simulink model "ROSCO"  (R2023a)
settings: Solver=ode4  StartTime=0.0  StopTime=TMax  FixedStep=simu.dt  RelTol=1e-3  EnableMultiTasking=on
undefined symbols (not defined in the file): A_total, Azimuth_list, B_total, Bd_total, C_total, D_total, Dd_total, DiscIntNeverNeededParam, F, n_FixFrameInputs, n_FixFrameOutputs, n_FixFrameStates2, n_RotTripletInputs, n_RotTripletOutputs, n_RotTripletStates2, new_seq_inp, new_seq_out, new_seq_states, OutList, Parameter, R, rpm2radps, simu, strmatch, uop_total, windspeed_list, wop_total, xop_total, yop_List_total
libraries: simulink x10
(part 3 of 5)

== system ROSCO/Monitor2/Cyclic Pitch controller/1P Cyclic Pitch Controller1/1P IPCDQ Filtering1/Moving 3P Notch Man Z/Moving 3P Filt Manual ==
  u : Inport
  rot speed (rad/s) : Inport  Port=2
  Den LPV : Subsystem
  Discrete Filter : DiscreteFilter  NumeratorSource=Input port  DenominatorSource=Input port  a0EqualsOne=on
      settings: InputPortMap=u0,p1,p3
  Num LPV : Subsystem
  Out1 : Outport  VectorParamsAs1DForOutWhenUnconnected=off
  wires:
  Den LPV/1(a) -> Discrete Filter/3
  rot speed (rad/s)/1 -> Num LPV/1(rot speed (rad/s)), Den LPV/1(rot speed (rad/s))
  Discrete Filter/1 -> Out1/1
  Num LPV/1(b) -> Discrete Filter/2
  u/1 -> Discrete Filter/1

== system ROSCO/Monitor2/Cyclic Pitch controller/1P Cyclic Pitch Controller1/1P IPCDQ Filtering1/Moving 6P Notch Man Y/Moving 6P Filt Manual ==
  u : Inport
  rot speed (rad/s) : Inport  Port=2
  Den LPV : Subsystem
  Discrete Filter : DiscreteFilter  NumeratorSource=Input port  DenominatorSource=Input port  a0EqualsOne=on
      settings: InputPortMap=u0,p1,p3
  Num LPV : Subsystem
  Out1 : Outport  VectorParamsAs1DForOutWhenUnconnected=off
  wires:
  Den LPV/1(a) -> Discrete Filter/3
  rot speed (rad/s)/1 -> Num LPV/1(rot speed (rad/s)), Den LPV/1(rot speed (rad/s))
  Discrete Filter/1 -> Out1/1
  Num LPV/1(b) -> Discrete Filter/2
  u/1 -> Discrete Filter/1

== system ROSCO/Monitor2/Cyclic Pitch controller/1P Cyclic Pitch Controller1/1P IPCDQ Filtering1/Moving 6P Notch Man Z/Moving 6P Filt Manual ==
  u : Inport
  rot speed (rad/s) : Inport  Port=2
  Den LPV : Subsystem
  Discrete Filter : DiscreteFilter  NumeratorSource=Input port  DenominatorSource=Input port  a0EqualsOne=on
      settings: InputPortMap=u0,p1,p3
  Num LPV : Subsystem
  Out1 : Outport  VectorParamsAs1DForOutWhenUnconnected=off
  wires:
  u/1 -> Discrete Filter/1
  Num LPV/1(b) -> Discrete Filter/2
  Discrete Filter/1 -> Out1/1
  rot speed (rad/s)/1 -> Den LPV/1(rot speed (rad/s)), Num LPV/1(rot speed (rad/s))
  Den LPV/1(a) -> Discrete Filter/3

== system ROSCO/Monitor2/Cyclic Pitch controller/1P Cyclic Pitch Controller1/M0 Signal Proc.1/Moving 1P Notch Man/Moving 1P Filt Manual ==
  u : Inport
  rot speed (rad/s) : Inport  Port=2
  Den LPV : Subsystem
  Discrete Filter : DiscreteFilter  NumeratorSource=Input port  DenominatorSource=Input port  a0EqualsOne=on
      settings: InputPortMap=u0,p1,p3
  Num LPV : Subsystem
  Out1 : Outport  VectorParamsAs1DForOutWhenUnconnected=off
  wires:
  Den LPV/1(a) -> Discrete Filter/3
  rot speed (rad/s)/1 -> Num LPV/1(rot speed (rad/s)), Den LPV/1(rot speed (rad/s))
  Discrete Filter/1 -> Out1/1
  Num LPV/1(b) -> Discrete Filter/2
  u/1 -> Discrete Filter/1

== system ROSCO/Monitor2/Cyclic Pitch controller/1P Cyclic Pitch Controller1/M0 Signal Proc.1/Moving 3P Notch Man/Moving 3P Filt Manual ==
  u : Inport
  rot speed (rad/s) : Inport  Port=2
  Den LPV : Subsystem
  Discrete Filter : DiscreteFilter  NumeratorSource=Input port  DenominatorSource=Input port  a0EqualsOne=on
      settings: InputPortMap=u0,p1,p3
  Num LPV : Subsystem
  Out1 : Outport  VectorParamsAs1DForOutWhenUnconnected=off
  wires:
  u/1 -> Discrete Filter/1
  Num LPV/1(b) -> Discrete Filter/2
  Discrete Filter/1 -> Out1/1
  rot speed (rad/s)/1 -> Den LPV/1(rot speed (rad/s)), Num LPV/1(rot speed (rad/s))
  Den LPV/1(a) -> Discrete Filter/3

== system ROSCO/Monitor2/Cyclic Pitch controller/2P Cyclic Pitch Controller2/1P IPCDQ Filtering1/Moving 3P Notch Man Y/Moving 3P Filt Manual ==
  u : Inport
  rot speed (rad/s) : Inport  Port=2
  Den LPV : Subsystem
  Discrete Filter : DiscreteFilter  NumeratorSource=Input port  DenominatorSource=Input port  a0EqualsOne=on
      settings: InputPortMap=u0,p1,p3
  Num LPV : Subsystem
  Out1 : Outport  VectorParamsAs1DForOutWhenUnconnected=off
  wires:
  u/1 -> Discrete Filter/1
  Num LPV/1(b) -> Discrete Filter/2
  Discrete Filter/1 -> Out1/1
  rot speed (rad/s)/1 -> Den LPV/1(rot speed (rad/s)), Num LPV/1(rot speed (rad/s))
  Den LPV/1(a) -> Discrete Filter/3

== system ROSCO/Monitor2/Cyclic Pitch controller/2P Cyclic Pitch Controller2/1P IPCDQ Filtering1/Moving 3P Notch Man Z/Moving 3P Filt Manual ==
  u : Inport
  rot speed (rad/s) : Inport  Port=2
  Den LPV : Subsystem
  Discrete Filter : DiscreteFilter  NumeratorSource=Input port  DenominatorSource=Input port  a0EqualsOne=on
      settings: InputPortMap=u0,p1,p3
  Num LPV : Subsystem
  Out1 : Outport  VectorParamsAs1DForOutWhenUnconnected=off
  wires:
  Den LPV/1(a) -> Discrete Filter/3
  rot speed (rad/s)/1 -> Num LPV/1(rot speed (rad/s)), Den LPV/1(rot speed (rad/s))
  Discrete Filter/1 -> Out1/1
  Num LPV/1(b) -> Discrete Filter/2
  u/1 -> Discrete Filter/1

== system ROSCO/Monitor2/Cyclic Pitch controller/2P Cyclic Pitch Controller2/1P IPCDQ Filtering1/Moving 6P Notch Man Y/Moving 6P Filt Manual ==
  u : Inport
  rot speed (rad/s) : Inport  Port=2
  Den LPV : Subsystem
  Discrete Filter : DiscreteFilter  NumeratorSource=Input port  DenominatorSource=Input port  a0EqualsOne=on
      settings: InputPortMap=u0,p1,p3
  Num LPV : Subsystem
  Out1 : Outport  VectorParamsAs1DForOutWhenUnconnected=off
  wires:
  Den LPV/1(a) -> Discrete Filter/3
  rot speed (rad/s)/1 -> Num LPV/1(rot speed (rad/s)), Den LPV/1(rot speed (rad/s))
  Discrete Filter/1 -> Out1/1
  Num LPV/1(b) -> Discrete Filter/2
  u/1 -> Discrete Filter/1

== system ROSCO/Monitor2/Cyclic Pitch controller/2P Cyclic Pitch Controller2/1P IPCDQ Filtering1/Moving 6P Notch Man Z/Moving 6P Filt Manual ==
  u : Inport
  rot speed (rad/s) : Inport  Port=2
  Den LPV : Subsystem
  Discrete Filter : DiscreteFilter  NumeratorSource=Input port  DenominatorSource=Input port  a0EqualsOne=on
      settings: InputPortMap=u0,p1,p3
  Num LPV : Subsystem
  Out1 : Outport  VectorParamsAs1DForOutWhenUnconnected=off
  wires:
  u/1 -> Discrete Filter/1
  Num LPV/1(b) -> Discrete Filter/2
  Discrete Filter/1 -> Out1/1
  rot speed (rad/s)/1 -> Den LPV/1(rot speed (rad/s)), Num LPV/1(rot speed (rad/s))
  Den LPV/1(a) -> Discrete Filter/3

== system ROSCO/Monitor2/Cyclic Pitch controller/2P Cyclic Pitch Controller2/M0 Signal Proc.1/Moving 1P Notch Man/Moving 1P Filt Manual ==
  u : Inport
  rot speed (rad/s) : Inport  Port=2
  Den LPV : Subsystem
  Discrete Filter : DiscreteFilter  NumeratorSource=Input port  DenominatorSource=Input port  a0EqualsOne=on
      settings: InputPortMap=u0,p1,p3
  Num LPV : Subsystem
  Out1 : Outport  VectorParamsAs1DForOutWhenUnconnected=off
  wires:
  Den LPV/1(a) -> Discrete Filter/3
  rot speed (rad/s)/1 -> Num LPV/1(rot speed (rad/s)), Den LPV/1(rot speed (rad/s))
  Discrete Filter/1 -> Out1/1
  Num LPV/1(b) -> Discrete Filter/2
  u/1 -> Discrete Filter/1

== system ROSCO/Monitor2/Cyclic Pitch controller/2P Cyclic Pitch Controller2/M0 Signal Proc.1/Moving 3P Notch Man/Moving 3P Filt Manual ==
  u : Inport
  rot speed (rad/s) : Inport  Port=2
  Den LPV : Subsystem
  Discrete Filter : DiscreteFilter  NumeratorSource=Input port  DenominatorSource=Input port  a0EqualsOne=on
      settings: InputPortMap=u0,p1,p3
  Num LPV : Subsystem
  Out1 : Outport  VectorParamsAs1DForOutWhenUnconnected=off
  wires:
  u/1 -> Discrete Filter/1
  Num LPV/1(b) -> Discrete Filter/2
  Discrete Filter/1 -> Out1/1
  rot speed (rad/s)/1 -> Den LPV/1(rot speed (rad/s)), Num LPV/1(rot speed (rad/s))
  Den LPV/1(a) -> Discrete Filter/3

== system ROSCO/Monitor2/Cyclic Pitch controller/1P Cyclic Pitch Controller1/1P IPCDQ Filtering1/Moving 3P Notch Man Y/Moving 3P Filt Manual/Den LPV ==
  rot speed (rad/s) : Inport
  1-D Lookup Table : Lookup_n-D  NumberOfTableDimensions=1  BreakpointsForDimension1=Parameter.Control.cIPC.PSM0_NF_3P.om_3P  BeginIndexSearchUsingPreviousIndexResult=on  Table=Parameter.Control.cIPC.PSM0_NF_3P.a_2  ExtrapMethod=Clip  InternalRulePriority=Speed  RndMeth=Simplest
  1-D Lookup Table1 : Lookup_n-D  NumberOfTableDimensions=1  BreakpointsForDimension1=Parameter.Control.cIPC.PSM0_NF_3P.om_3P  BeginIndexSearchUsingPreviousIndexResult=on  Table=Parameter.Control.cIPC.PSM0_NF_3P.a_1  ExtrapMethod=Clip  InternalRulePriority=Speed  RndMeth=Simplest
  1-D Lookup Table2 : Lookup_n-D  NumberOfTableDimensions=1  BreakpointsForDimension1=Parameter.Control.cIPC.PSM0_NF_3P.om_3P  BeginIndexSearchUsingPreviousIndexResult=on  Table=Parameter.Control.cIPC.PSM0_NF_3P.a_0  ExtrapMethod=Clip  InternalRulePriority=Speed  RndMeth=Simplest
  Mux : Mux  Inputs=3
  a : Outport  VectorParamsAs1DForOutWhenUnconnected=off
  wires:
  1-D Lookup Table/1 -> Mux/1
  1-D Lookup Table1/1 -> Mux/2
  Mux/1 -> a/1
  rot speed (rad/s)/1 -> 1-D Lookup Table2/1, 1-D Lookup Table/1, 1-D Lookup Table1/1
  1-D Lookup Table2/1 -> Mux/3

== system ROSCO/Monitor2/Cyclic Pitch controller/1P Cyclic Pitch Controller1/1P IPCDQ Filtering1/Moving 3P Notch Man Y/Moving 3P Filt Manual/Num LPV ==
  rot speed (rad/s) : Inport
  1-D Lookup Table : Lookup_n-D  NumberOfTableDimensions=1  BreakpointsForDimension1=Parameter.Control.cIPC.PSM0_NF_3P.om_3P  BeginIndexSearchUsingPreviousIndexResult=on  Table=Parameter.Control.cIPC.PSM0_NF_3P.b_2  ExtrapMethod=Clip  InternalRulePriority=Speed  RndMeth=Simplest
  1-D Lookup Table1 : Lookup_n-D  NumberOfTableDimensions=1  BreakpointsForDimension1=Parameter.Control.cIPC.PSM0_NF_3P.om_3P  BeginIndexSearchUsingPreviousIndexResult=on  Table=Parameter.Control.cIPC.PSM0_NF_3P.b_1  ExtrapMethod=Clip  InternalRulePriority=Speed  RndMeth=Simplest
  1-D Lookup Table2 : Lookup_n-D  NumberOfTableDimensions=1  BreakpointsForDimension1=Parameter.Control.cIPC.PSM0_NF_3P.om_3P  BeginIndexSearchUsingPreviousIndexResult=on  Table=Parameter.Control.cIPC.PSM0_NF_3P.b_0  ExtrapMethod=Clip  InternalRulePriority=Speed  RndMeth=Simplest
  Mux : Mux  Inputs=3
  b : Outport  VectorParamsAs1DForOutWhenUnconnected=off
  wires:
  1-D Lookup Table2/1 -> Mux/3
  rot speed (rad/s)/1 -> 1-D Lookup Table1/1, 1-D Lookup Table/1, 1-D Lookup Table2/1
  Mux/1 -> b/1
  1-D Lookup Table1/1 -> Mux/2
  1-D Lookup Table/1 -> Mux/1

== system ROSCO/Monitor2/Cyclic Pitch controller/1P Cyclic Pitch Controller1/1P IPCDQ Filtering1/Moving 3P Notch Man Z/Moving 3P Filt Manual/Den LPV ==
  rot speed (rad/s) : Inport
  1-D Lookup Table : Lookup_n-D  NumberOfTableDimensions=1  BreakpointsForDimension1=Parameter.Control.cIPC.PSM0_NF_3P.om_3P  BeginIndexSearchUsingPreviousIndexResult=on  Table=Parameter.Control.cIPC.PSM0_NF_3P.a_2  ExtrapMethod=Clip  InternalRulePriority=Speed  RndMeth=Simplest
  1-D Lookup Table1 : Lookup_n-D  NumberOfTableDimensions=1  BreakpointsForDimension1=Parameter.Control.cIPC.PSM0_NF_3P.om_3P  BeginIndexSearchUsingPreviousIndexResult=on  Table=Parameter.Control.cIPC.PSM0_NF_3P.a_1  ExtrapMethod=Clip  InternalRulePriority=Speed  RndMeth=Simplest
  1-D Lookup Table2 : Lookup_n-D  NumberOfTableDimensions=1  BreakpointsForDimension1=Parameter.Control.cIPC.PSM0_NF_3P.om_3P  BeginIndexSearchUsingPreviousIndexResult=on  Table=Parameter.Control.cIPC.PSM0_NF_3P.a_0  ExtrapMethod=Clip  InternalRulePriority=Speed  RndMeth=Simplest
  Mux : Mux  Inputs=3
  a : Outport  VectorParamsAs1DForOutWhenUnconnected=off
  wires:
  1-D Lookup Table2/1 -> Mux/3
  rot speed (rad/s)/1 -> 1-D Lookup Table1/1, 1-D Lookup Table/1, 1-D Lookup Table2/1
  Mux/1 -> a/1
  1-D Lookup Table1/1 -> Mux/2
  1-D Lookup Table/1 -> Mux/1

== system ROSCO/Monitor2/Cyclic Pitch controller/1P Cyclic Pitch Controller1/1P IPCDQ Filtering1/Moving 3P Notch Man Z/Moving 3P Filt Manual/Num LPV ==
  rot speed (rad/s) : Inport
  1-D Lookup Table : Lookup_n-D  NumberOfTableDimensions=1  BreakpointsForDimension1=Parameter.Control.cIPC.PSM0_NF_3P.om_3P  BeginIndexSearchUsingPreviousIndexResult=on  Table=Parameter.Control.cIPC.PSM0_NF_3P.b_2  ExtrapMethod=Clip  InternalRulePriority=Speed  RndMeth=Simplest
  1-D Lookup Table1 : Lookup_n-D  NumberOfTableDimensions=1  BreakpointsForDimension1=Parameter.Control.cIPC.PSM0_NF_3P.om_3P  BeginIndexSearchUsingPreviousIndexResult=on  Table=Parameter.Control.cIPC.PSM0_NF_3P.b_1  ExtrapMethod=Clip  InternalRulePriority=Speed  RndMeth=Simplest
  1-D Lookup Table2 : Lookup_n-D  NumberOfTableDimensions=1  BreakpointsForDimension1=Parameter.Control.cIPC.PSM0_NF_3P.om_3P  BeginIndexSearchUsingPreviousIndexResult=on  Table=Parameter.Control.cIPC.PSM0_NF_3P.b_0  ExtrapMethod=Clip  InternalRulePriority=Speed  RndMeth=Simplest
  Mux : Mux  Inputs=3
  b : Outport  VectorParamsAs1DForOutWhenUnconnected=off
  wires:
  1-D Lookup Table/1 -> Mux/1
  1-D Lookup Table1/1 -> Mux/2
  Mux/1 -> b/1
  rot speed (rad/s)/1 -> 1-D Lookup Table2/1, 1-D Lookup Table/1, 1-D Lookup Table1/1
  1-D Lookup Table2/1 -> Mux/3

== system ROSCO/Monitor2/Cyclic Pitch controller/1P Cyclic Pitch Controller1/1P IPCDQ Filtering1/Moving 6P Notch Man Y/Moving 6P Filt Manual/Den LPV ==
  rot speed (rad/s) : Inport
  1-D Lookup Table : Lookup_n-D  NumberOfTableDimensions=1  BreakpointsForDimension1=Parameter.Control.cIPC.PSM0_NF_6P.om_6P  BeginIndexSearchUsingPreviousIndexResult=on  Table=Parameter.Control.cIPC.PSM0_NF_6P.a_2  ExtrapMethod=Clip  InternalRulePriority=Speed  RndMeth=Simplest
  1-D Lookup Table1 : Lookup_n-D  NumberOfTableDimensions=1  BreakpointsForDimension1=Parameter.Control.cIPC.PSM0_NF_6P.om_6P  BeginIndexSearchUsingPreviousIndexResult=on  Table=Parameter.Control.cIPC.PSM0_NF_6P.a_1  ExtrapMethod=Clip  InternalRulePriority=Speed  RndMeth=Simplest
  1-D Lookup Table2 : Lookup_n-D  NumberOfTableDimensions=1  BreakpointsForDimension1=Parameter.Control.cIPC.PSM0_NF_6P.om_6P  BeginIndexSearchUsingPreviousIndexResult=on  Table=Parameter.Control.cIPC.PSM0_NF_6P.a_0  ExtrapMethod=Clip  InternalRulePriority=Speed  RndMeth=Simplest
  Mux : Mux  Inputs=3
  a : Outport  VectorParamsAs1DForOutWhenUnconnected=off
  wires:
  1-D Lookup Table2/1 -> Mux/3
  rot speed (rad/s)/1 -> 1-D Lookup Table1/1, 1-D Lookup Table/1, 1-D Lookup Table2/1
  Mux/1 -> a/1
  1-D Lookup Table1/1 -> Mux/2
  1-D Lookup Table/1 -> Mux/1

== system ROSCO/Monitor2/Cyclic Pitch controller/1P Cyclic Pitch Controller1/1P IPCDQ Filtering1/Moving 6P Notch Man Y/Moving 6P Filt Manual/Num LPV ==
  rot speed (rad/s) : Inport
  1-D Lookup Table : Lookup_n-D  NumberOfTableDimensions=1  BreakpointsForDimension1=Parameter.Control.cIPC.PSM0_NF_6P.om_6P  BeginIndexSearchUsingPreviousIndexResult=on  Table=Parameter.Control.cIPC.PSM0_NF_6P.b_2  ExtrapMethod=Clip  InternalRulePriority=Speed  RndMeth=Simplest
  1-D Lookup Table1 : Lookup_n-D  NumberOfTableDimensions=1  BreakpointsForDimension1=Parameter.Control.cIPC.PSM0_NF_6P.om_6P  BeginIndexSearchUsingPreviousIndexResult=on  Table=Parameter.Control.cIPC.PSM0_NF_6P.b_1  ExtrapMethod=Clip  InternalRulePriority=Speed  RndMeth=Simplest
  1-D Lookup Table2 : Lookup_n-D  NumberOfTableDimensions=1  BreakpointsForDimension1=Parameter.Control.cIPC.PSM0_NF_6P.om_6P  BeginIndexSearchUsingPreviousIndexResult=on  Table=Parameter.Control.cIPC.PSM0_NF_6P.b_0  ExtrapMethod=Clip  InternalRulePriority=Speed  RndMeth=Simplest
  Mux : Mux  Inputs=3
  b : Outport  VectorParamsAs1DForOutWhenUnconnected=off
  wires:
  1-D Lookup Table/1 -> Mux/1
  1-D Lookup Table1/1 -> Mux/2
  Mux/1 -> b/1
  rot speed (rad/s)/1 -> 1-D Lookup Table2/1, 1-D Lookup Table1/1, 1-D Lookup Table/1
  1-D Lookup Table2/1 -> Mux/3

== system ROSCO/Monitor2/Cyclic Pitch controller/1P Cyclic Pitch Controller1/1P IPCDQ Filtering1/Moving 6P Notch Man Z/Moving 6P Filt Manual/Den LPV ==
  rot speed (rad/s) : Inport
  1-D Lookup Table : Lookup_n-D  NumberOfTableDimensions=1  BreakpointsForDimension1=Parameter.Control.cIPC.PSM0_NF_6P.om_6P  BeginIndexSearchUsingPreviousIndexResult=on  Table=Parameter.Control.cIPC.PSM0_NF_6P.a_2  ExtrapMethod=Clip  InternalRulePriority=Speed  RndMeth=Simplest
  1-D Lookup Table1 : Lookup_n-D  NumberOfTableDimensions=1  BreakpointsForDimension1=Parameter.Control.cIPC.PSM0_NF_6P.om_6P  BeginIndexSearchUsingPreviousIndexResult=on  Table=Parameter.Control.cIPC.PSM0_NF_6P.a_1  ExtrapMethod=Clip  InternalRulePriority=Speed  RndMeth=Simplest
  1-D Lookup Table2 : Lookup_n-D  NumberOfTableDimensions=1  BreakpointsForDimension1=Parameter.Control.cIPC.PSM0_NF_6P.om_6P  BeginIndexSearchUsingPreviousIndexResult=on  Table=Parameter.Control.cIPC.PSM0_NF_6P.a_0  ExtrapMethod=Clip  InternalRulePriority=Speed  RndMeth=Simplest
  Mux : Mux  Inputs=3
  a : Outport  VectorParamsAs1DForOutWhenUnconnected=off
  wires:
  1-D Lookup Table/1 -> Mux/1
  1-D Lookup Table1/1 -> Mux/2
  Mux/1 -> a/1
  rot speed (rad/s)/1 -> 1-D Lookup Table2/1, 1-D Lookup Table/1, 1-D Lookup Table1/1
  1-D Lookup Table2/1 -> Mux/3

== system ROSCO/Monitor2/Cyclic Pitch controller/1P Cyclic Pitch Controller1/1P IPCDQ Filtering1/Moving 6P Notch Man Z/Moving 6P Filt Manual/Num LPV ==
  rot speed (rad/s) : Inport
  1-D Lookup Table : Lookup_n-D  NumberOfTableDimensions=1  BreakpointsForDimension1=Parameter.Control.cIPC.PSM0_NF_6P.om_6P  BeginIndexSearchUsingPreviousIndexResult=on  Table=Parameter.Control.cIPC.PSM0_NF_6P.b_2  ExtrapMethod=Clip  InternalRulePriority=Speed  RndMeth=Simplest
  1-D Lookup Table1 : Lookup_n-D  NumberOfTableDimensions=1  BreakpointsForDimension1=Parameter.Control.cIPC.PSM0_NF_6P.om_6P  BeginIndexSearchUsingPreviousIndexResult=on  Table=Parameter.Control.cIPC.PSM0_NF_6P.b_1  ExtrapMethod=Clip  InternalRulePriority=Speed  RndMeth=Simplest
  1-D Lookup Table2 : Lookup_n-D  NumberOfTableDimensions=1  BreakpointsForDimension1=Parameter.Control.cIPC.PSM0_NF_6P.om_6P  BeginIndexSearchUsingPreviousIndexResult=on  Table=Parameter.Control.cIPC.PSM0_NF_6P.b_0  ExtrapMethod=Clip  InternalRulePriority=Speed  RndMeth=Simplest
  Mux : Mux  Inputs=3
  b : Outport  VectorParamsAs1DForOutWhenUnconnected=off
  wires:
  1-D Lookup Table2/1 -> Mux/3
  rot speed (rad/s)/1 -> 1-D Lookup Table1/1, 1-D Lookup Table/1, 1-D Lookup Table2/1
  Mux/1 -> b/1
  1-D Lookup Table1/1 -> Mux/2
  1-D Lookup Table/1 -> Mux/1

== system ROSCO/Monitor2/Cyclic Pitch controller/1P Cyclic Pitch Controller1/M0 Signal Proc.1/Moving 1P Notch Man/Moving 1P Filt Manual/Den LPV ==
  rot speed (rad/s) : Inport
  1-D Lookup Table : Lookup_n-D  NumberOfTableDimensions=1  BreakpointsForDimension1=Parameter.Control.cIPC.PSM0_NF_1P.om_1P  BeginIndexSearchUsingPreviousIndexResult=on  Table=Parameter.Control.cIPC.PSM0_NF_1P.a_2  ExtrapMethod=Clip  InternalRulePriority=Speed  RndMeth=Simplest
  1-D Lookup Table1 : Lookup_n-D  NumberOfTableDimensions=1  BreakpointsForDimension1=Parameter.Control.cIPC.PSM0_NF_1P.om_1P  BeginIndexSearchUsingPreviousIndexResult=on  Table=Parameter.Control.cIPC.PSM0_NF_1P.a_1  ExtrapMethod=Clip  InternalRulePriority=Speed  RndMeth=Simplest
  1-D Lookup Table2 : Lookup_n-D  NumberOfTableDimensions=1  BreakpointsForDimension1=Parameter.Control.cIPC.PSM0_NF_1P.om_1P  BeginIndexSearchUsingPreviousIndexResult=on  Table=Parameter.Control.cIPC.PSM0_NF_1P.a_0  ExtrapMethod=Clip  InternalRulePriority=Speed  RndMeth=Simplest
  Mux : Mux  Inputs=3
  a : Outport  VectorParamsAs1DForOutWhenUnconnected=off
  wires:
  1-D Lookup Table2/1 -> Mux/3
  rot speed (rad/s)/1 -> 1-D Lookup Table1/1, 1-D Lookup Table/1, 1-D Lookup Table2/1
  Mux/1 -> a/1
  1-D Lookup Table1/1 -> Mux/2
  1-D Lookup Table/1 -> Mux/1

== system ROSCO/Monitor2/Cyclic Pitch controller/1P Cyclic Pitch Controller1/M0 Signal Proc.1/Moving 1P Notch Man/Moving 1P Filt Manual/Num LPV ==
  rot speed (rad/s) : Inport
  1-D Lookup Table : Lookup_n-D  NumberOfTableDimensions=1  BreakpointsForDimension1=Parameter.Control.cIPC.PSM0_NF_1P.om_1P  BeginIndexSearchUsingPreviousIndexResult=on  Table=Parameter.Control.cIPC.PSM0_NF_1P.b_2  ExtrapMethod=Clip  InternalRulePriority=Speed  RndMeth=Simplest
  1-D Lookup Table1 : Lookup_n-D  NumberOfTableDimensions=1  BreakpointsForDimension1=Parameter.Control.cIPC.PSM0_NF_1P.om_1P  BeginIndexSearchUsingPreviousIndexResult=on  Table=Parameter.Control.cIPC.PSM0_NF_1P.b_1  ExtrapMethod=Clip  InternalRulePriority=Speed  RndMeth=Simplest
  1-D Lookup Table2 : Lookup_n-D  NumberOfTableDimensions=1  BreakpointsForDimension1=Parameter.Control.cIPC.PSM0_NF_1P.om_1P  BeginIndexSearchUsingPreviousIndexResult=on  Table=Parameter.Control.cIPC.PSM0_NF_1P.b_0  ExtrapMethod=Clip  InternalRulePriority=Speed  RndMeth=Simplest
  Mux : Mux  Inputs=3
  b : Outport  VectorParamsAs1DForOutWhenUnconnected=off
  wires:
  1-D Lookup Table/1 -> Mux/1
  1-D Lookup Table1/1 -> Mux/2
  Mux/1 -> b/1
  rot speed (rad/s)/1 -> 1-D Lookup Table2/1, 1-D Lookup Table/1, 1-D Lookup Table1/1
  1-D Lookup Table2/1 -> Mux/3

== system ROSCO/Monitor2/Cyclic Pitch controller/1P Cyclic Pitch Controller1/M0 Signal Proc.1/Moving 3P Notch Man/Moving 3P Filt Manual/Den LPV ==
  rot speed (rad/s) : Inport
  1-D Lookup Table : Lookup_n-D  NumberOfTableDimensions=1  BreakpointsForDimension1=Parameter.Control.cIPC.PSM0_NF_3P.om_3P  BeginIndexSearchUsingPreviousIndexResult=on  Table=Parameter.Control.cIPC.PSM0_NF_3P.a_2  ExtrapMethod=Clip  InternalRulePriority=Speed  RndMeth=Simplest
  1-D Lookup Table1 : Lookup_n-D  NumberOfTableDimensions=1  BreakpointsForDimension1=Parameter.Control.cIPC.PSM0_NF_3P.om_3P  BeginIndexSearchUsingPreviousIndexResult=on  Table=Parameter.Control.cIPC.PSM0_NF_3P.a_1  ExtrapMethod=Clip  InternalRulePriority=Speed  RndMeth=Simplest
  1-D Lookup Table2 : Lookup_n-D  NumberOfTableDimensions=1  BreakpointsForDimension1=Parameter.Control.cIPC.PSM0_NF_3P.om_3P  BeginIndexSearchUsingPreviousIndexResult=on  Table=Parameter.Control.cIPC.PSM0_NF_3P.a_0  ExtrapMethod=Clip  InternalRulePriority=Speed  RndMeth=Simplest
  Mux : Mux  Inputs=3
  a : Outport  VectorParamsAs1DForOutWhenUnconnected=off
  wires:
  1-D Lookup Table/1 -> Mux/1
  1-D Lookup Table1/1 -> Mux/2
  Mux/1 -> a/1
  rot speed (rad/s)/1 -> 1-D Lookup Table2/1, 1-D Lookup Table/1, 1-D Lookup Table1/1
  1-D Lookup Table2/1 -> Mux/3

== system ROSCO/Monitor2/Cyclic Pitch controller/1P Cyclic Pitch Controller1/M0 Signal Proc.1/Moving 3P Notch Man/Moving 3P Filt Manual/Num LPV ==
  rot speed (rad/s) : Inport
  1-D Lookup Table : Lookup_n-D  NumberOfTableDimensions=1  BreakpointsForDimension1=Parameter.Control.cIPC.PSM0_NF_3P.om_3P  BeginIndexSearchUsingPreviousIndexResult=on  Table=Parameter.Control.cIPC.PSM0_NF_3P.b_2  ExtrapMethod=Clip  InternalRulePriority=Speed  RndMeth=Simplest
  1-D Lookup Table1 : Lookup_n-D  NumberOfTableDimensions=1  BreakpointsForDimension1=Parameter.Control.cIPC.PSM0_NF_3P.om_3P  BeginIndexSearchUsingPreviousIndexResult=on  Table=Parameter.Control.cIPC.PSM0_NF_3P.b_1  ExtrapMethod=Clip  InternalRulePriority=Speed  RndMeth=Simplest
  1-D Lookup Table2 : Lookup_n-D  NumberOfTableDimensions=1  BreakpointsForDimension1=Parameter.Control.cIPC.PSM0_NF_3P.om_3P  BeginIndexSearchUsingPreviousIndexResult=on  Table=Parameter.Control.cIPC.PSM0_NF_3P.b_0  ExtrapMethod=Clip  InternalRulePriority=Speed  RndMeth=Simplest
  Mux : Mux  Inputs=3
  b : Outport  VectorParamsAs1DForOutWhenUnconnected=off
  wires:
  1-D Lookup Table2/1 -> Mux/3
  rot speed (rad/s)/1 -> 1-D Lookup Table1/1, 1-D Lookup Table/1, 1-D Lookup Table2/1
  Mux/1 -> b/1
  1-D Lookup Table1/1 -> Mux/2
  1-D Lookup Table/1 -> Mux/1

== system ROSCO/Monitor2/Cyclic Pitch controller/2P Cyclic Pitch Controller2/1P IPCDQ Filtering1/Moving 3P Notch Man Y/Moving 3P Filt Manual/Den LPV ==
  rot speed (rad/s) : Inport
  1-D Lookup Table : Lookup_n-D  NumberOfTableDimensions=1  BreakpointsForDimension1=Parameter.Control.cIPC.PSM0_NF_3P.om_3P  BeginIndexSearchUsingPreviousIndexResult=on  Table=Parameter.Control.cIPC.PSM0_NF_3P.a_2  ExtrapMethod=Clip  InternalRulePriority=Speed  RndMeth=Simplest
  1-D Lookup Table1 : Lookup_n-D  NumberOfTableDimensions=1  BreakpointsForDimension1=Parameter.Control.cIPC.PSM0_NF_3P.om_3P  BeginIndexSearchUsingPreviousIndexResult=on  Table=Parameter.Control.cIPC.PSM0_NF_3P.a_1  ExtrapMethod=Clip  InternalRulePriority=Speed  RndMeth=Simplest
  1-D Lookup Table2 : Lookup_n-D  NumberOfTableDimensions=1  BreakpointsForDimension1=Parameter.Control.cIPC.PSM0_NF_3P.om_3P  BeginIndexSearchUsingPreviousIndexResult=on  Table=Parameter.Control.cIPC.PSM0_NF_3P.a_0  ExtrapMethod=Clip  InternalRulePriority=Speed  RndMeth=Simplest
  Mux : Mux  Inputs=3
  a : Outport  VectorParamsAs1DForOutWhenUnconnected=off
  wires:
  1-D Lookup Table/1 -> Mux/1
  1-D Lookup Table1/1 -> Mux/2
  Mux/1 -> a/1
  rot speed (rad/s)/1 -> 1-D Lookup Table2/1, 1-D Lookup Table/1, 1-D Lookup Table1/1
  1-D Lookup Table2/1 -> Mux/3

== system ROSCO/Monitor2/Cyclic Pitch controller/2P Cyclic Pitch Controller2/1P IPCDQ Filtering1/Moving 3P Notch Man Y/Moving 3P Filt Manual/Num LPV ==
  rot speed (rad/s) : Inport
  1-D Lookup Table : Lookup_n-D  NumberOfTableDimensions=1  BreakpointsForDimension1=Parameter.Control.cIPC.PSM0_NF_3P.om_3P  BeginIndexSearchUsingPreviousIndexResult=on  Table=Parameter.Control.cIPC.PSM0_NF_3P.b_2  ExtrapMethod=Clip  InternalRulePriority=Speed  RndMeth=Simplest
  1-D Lookup Table1 : Lookup_n-D  NumberOfTableDimensions=1  BreakpointsForDimension1=Parameter.Control.cIPC.PSM0_NF_3P.om_3P  BeginIndexSearchUsingPreviousIndexResult=on  Table=Parameter.Control.cIPC.PSM0_NF_3P.b_1  ExtrapMethod=Clip  InternalRulePriority=Speed  RndMeth=Simplest
  1-D Lookup Table2 : Lookup_n-D  NumberOfTableDimensions=1  BreakpointsForDimension1=Parameter.Control.cIPC.PSM0_NF_3P.om_3P  BeginIndexSearchUsingPreviousIndexResult=on  Table=Parameter.Control.cIPC.PSM0_NF_3P.b_0  ExtrapMethod=Clip  InternalRulePriority=Speed  RndMeth=Simplest
  Mux : Mux  Inputs=3
  b : Outport  VectorParamsAs1DForOutWhenUnconnected=off
  wires:
  1-D Lookup Table2/1 -> Mux/3
  rot speed (rad/s)/1 -> 1-D Lookup Table1/1, 1-D Lookup Table/1, 1-D Lookup Table2/1
  Mux/1 -> b/1
  1-D Lookup Table1/1 -> Mux/2
  1-D Lookup Table/1 -> Mux/1

== system ROSCO/Monitor2/Cyclic Pitch controller/2P Cyclic Pitch Controller2/1P IPCDQ Filtering1/Moving 3P Notch Man Z/Moving 3P Filt Manual/Den LPV ==
  rot speed (rad/s) : Inport
  1-D Lookup Table : Lookup_n-D  NumberOfTableDimensions=1  BreakpointsForDimension1=Parameter.Control.cIPC.PSM0_NF_3P.om_3P  BeginIndexSearchUsingPreviousIndexResult=on  Table=Parameter.Control.cIPC.PSM0_NF_3P.a_2  ExtrapMethod=Clip  InternalRulePriority=Speed  RndMeth=Simplest
  1-D Lookup Table1 : Lookup_n-D  NumberOfTableDimensions=1  BreakpointsForDimension1=Parameter.Control.cIPC.PSM0_NF_3P.om_3P  BeginIndexSearchUsingPreviousIndexResult=on  Table=Parameter.Control.cIPC.PSM0_NF_3P.a_1  ExtrapMethod=Clip  InternalRulePriority=Speed  RndMeth=Simplest
  1-D Lookup Table2 : Lookup_n-D  NumberOfTableDimensions=1  BreakpointsForDimension1=Parameter.Control.cIPC.PSM0_NF_3P.om_3P  BeginIndexSearchUsingPreviousIndexResult=on  Table=Parameter.Control.cIPC.PSM0_NF_3P.a_0  ExtrapMethod=Clip  InternalRulePriority=Speed  RndMeth=Simplest
  Mux : Mux  Inputs=3
  a : Outport  VectorParamsAs1DForOutWhenUnconnected=off
  wires:
  1-D Lookup Table2/1 -> Mux/3
  rot speed (rad/s)/1 -> 1-D Lookup Table1/1, 1-D Lookup Table/1, 1-D Lookup Table2/1
  Mux/1 -> a/1
  1-D Lookup Table1/1 -> Mux/2
  1-D Lookup Table/1 -> Mux/1

== system ROSCO/Monitor2/Cyclic Pitch controller/2P Cyclic Pitch Controller2/1P IPCDQ Filtering1/Moving 3P Notch Man Z/Moving 3P Filt Manual/Num LPV ==
  rot speed (rad/s) : Inport
  1-D Lookup Table : Lookup_n-D  NumberOfTableDimensions=1  BreakpointsForDimension1=Parameter.Control.cIPC.PSM0_NF_3P.om_3P  BeginIndexSearchUsingPreviousIndexResult=on  Table=Parameter.Control.cIPC.PSM0_NF_3P.b_2  ExtrapMethod=Clip  InternalRulePriority=Speed  RndMeth=Simplest
  1-D Lookup Table1 : Lookup_n-D  NumberOfTableDimensions=1  BreakpointsForDimension1=Parameter.Control.cIPC.PSM0_NF_3P.om_3P  BeginIndexSearchUsingPreviousIndexResult=on  Table=Parameter.Control.cIPC.PSM0_NF_3P.b_1  ExtrapMethod=Clip  InternalRulePriority=Speed  RndMeth=Simplest
  1-D Lookup Table2 : Lookup_n-D  NumberOfTableDimensions=1  BreakpointsForDimension1=Parameter.Control.cIPC.PSM0_NF_3P.om_3P  BeginIndexSearchUsingPreviousIndexResult=on  Table=Parameter.Control.cIPC.PSM0_NF_3P.b_0  ExtrapMethod=Clip  InternalRulePriority=Speed  RndMeth=Simplest
  Mux : Mux  Inputs=3
  b : Outport  VectorParamsAs1DForOutWhenUnconnected=off
  wires:
  1-D Lookup Table/1 -> Mux/1
  1-D Lookup Table1/1 -> Mux/2
  Mux/1 -> b/1
  rot speed (rad/s)/1 -> 1-D Lookup Table2/1, 1-D Lookup Table/1, 1-D Lookup Table1/1
  1-D Lookup Table2/1 -> Mux/3

== system ROSCO/Monitor2/Cyclic Pitch controller/2P Cyclic Pitch Controller2/1P IPCDQ Filtering1/Moving 6P Notch Man Y/Moving 6P Filt Manual/Den LPV ==
  rot speed (rad/s) : Inport
  1-D Lookup Table : Lookup_n-D  NumberOfTableDimensions=1  BreakpointsForDimension1=Parameter.Control.cIPC.PSM0_NF_6P.om_6P  BeginIndexSearchUsingPreviousIndexResult=on  Table=Parameter.Control.cIPC.PSM0_NF_6P.a_2  ExtrapMethod=Clip  InternalRulePriority=Speed  RndMeth=Simplest
  1-D Lookup Table1 : Lookup_n-D  NumberOfTableDimensions=1  BreakpointsForDimension1=Parameter.Control.cIPC.PSM0_NF_6P.om_6P  BeginIndexSearchUsingPreviousIndexResult=on  Table=Parameter.Control.cIPC.PSM0_NF_6P.a_1  ExtrapMethod=Clip  InternalRulePriority=Speed  RndMeth=Simplest
  1-D Lookup Table2 : Lookup_n-D  NumberOfTableDimensions=1  BreakpointsForDimension1=Parameter.Control.cIPC.PSM0_NF_6P.om_6P  BeginIndexSearchUsingPreviousIndexResult=on  Table=Parameter.Control.cIPC.PSM0_NF_6P.a_0  ExtrapMethod=Clip  InternalRulePriority=Speed  RndMeth=Simplest
  Mux : Mux  Inputs=3
  a : Outport  VectorParamsAs1DForOutWhenUnconnected=off
  wires:
  1-D Lookup Table2/1 -> Mux/3
  rot speed (rad/s)/1 -> 1-D Lookup Table1/1, 1-D Lookup Table/1, 1-D Lookup Table2/1
  Mux/1 -> a/1
  1-D Lookup Table1/1 -> Mux/2
  1-D Lookup Table/1 -> Mux/1

== system ROSCO/Monitor2/Cyclic Pitch controller/2P Cyclic Pitch Controller2/1P IPCDQ Filtering1/Moving 6P Notch Man Y/Moving 6P Filt Manual/Num LPV ==
  rot speed (rad/s) : Inport
  1-D Lookup Table : Lookup_n-D  NumberOfTableDimensions=1  BreakpointsForDimension1=Parameter.Control.cIPC.PSM0_NF_6P.om_6P  BeginIndexSearchUsingPreviousIndexResult=on  Table=Parameter.Control.cIPC.PSM0_NF_6P.b_2  ExtrapMethod=Clip  InternalRulePriority=Speed  RndMeth=Simplest
  1-D Lookup Table1 : Lookup_n-D  NumberOfTableDimensions=1  BreakpointsForDimension1=Parameter.Control.cIPC.PSM0_NF_6P.om_6P  BeginIndexSearchUsingPreviousIndexResult=on  Table=Parameter.Control.cIPC.PSM0_NF_6P.b_1  ExtrapMethod=Clip  InternalRulePriority=Speed  RndMeth=Simplest
  1-D Lookup Table2 : Lookup_n-D  NumberOfTableDimensions=1  BreakpointsForDimension1=Parameter.Control.cIPC.PSM0_NF_6P.om_6P  BeginIndexSearchUsingPreviousIndexResult=on  Table=Parameter.Control.cIPC.PSM0_NF_6P.b_0  ExtrapMethod=Clip  InternalRulePriority=Speed  RndMeth=Simplest
  Mux : Mux  Inputs=3
  b : Outport  VectorParamsAs1DForOutWhenUnconnected=off
  wires:
  1-D Lookup Table/1 -> Mux/1
  1-D Lookup Table1/1 -> Mux/2
  Mux/1 -> b/1
  rot speed (rad/s)/1 -> 1-D Lookup Table2/1, 1-D Lookup Table1/1, 1-D Lookup Table/1
  1-D Lookup Table2/1 -> Mux/3

== system ROSCO/Monitor2/Cyclic Pitch controller/2P Cyclic Pitch Controller2/1P IPCDQ Filtering1/Moving 6P Notch Man Z/Moving 6P Filt Manual/Den LPV ==
  rot speed (rad/s) : Inport
  1-D Lookup Table : Lookup_n-D  NumberOfTableDimensions=1  BreakpointsForDimension1=Parameter.Control.cIPC.PSM0_NF_6P.om_6P  BeginIndexSearchUsingPreviousIndexResult=on  Table=Parameter.Control.cIPC.PSM0_NF_6P.a_2  ExtrapMethod=Clip  InternalRulePriority=Speed  RndMeth=Simplest
  1-D Lookup Table1 : Lookup_n-D  NumberOfTableDimensions=1  BreakpointsForDimension1=Parameter.Control.cIPC.PSM0_NF_6P.om_6P  BeginIndexSearchUsingPreviousIndexResult=on  Table=Parameter.Control.cIPC.PSM0_NF_6P.a_1  ExtrapMethod=Clip  InternalRulePriority=Speed  RndMeth=Simplest
  1-D Lookup Table2 : Lookup_n-D  NumberOfTableDimensions=1  BreakpointsForDimension1=Parameter.Control.cIPC.PSM0_NF_6P.om_6P  BeginIndexSearchUsingPreviousIndexResult=on  Table=Parameter.Control.cIPC.PSM0_NF_6P.a_0  ExtrapMethod=Clip  InternalRulePriority=Speed  RndMeth=Simplest
  Mux : Mux  Inputs=3
  a : Outport  VectorParamsAs1DForOutWhenUnconnected=off
  wires:
  1-D Lookup Table/1 -> Mux/1
  1-D Lookup Table1/1 -> Mux/2
  Mux/1 -> a/1
  rot speed (rad/s)/1 -> 1-D Lookup Table2/1, 1-D Lookup Table/1, 1-D Lookup Table1/1
  1-D Lookup Table2/1 -> Mux/3

== system ROSCO/Monitor2/Cyclic Pitch controller/2P Cyclic Pitch Controller2/1P IPCDQ Filtering1/Moving 6P Notch Man Z/Moving 6P Filt Manual/Num LPV ==
  rot speed (rad/s) : Inport
  1-D Lookup Table : Lookup_n-D  NumberOfTableDimensions=1  BreakpointsForDimension1=Parameter.Control.cIPC.PSM0_NF_6P.om_6P  BeginIndexSearchUsingPreviousIndexResult=on  Table=Parameter.Control.cIPC.PSM0_NF_6P.b_2  ExtrapMethod=Clip  InternalRulePriority=Speed  RndMeth=Simplest
  1-D Lookup Table1 : Lookup_n-D  NumberOfTableDimensions=1  BreakpointsForDimension1=Parameter.Control.cIPC.PSM0_NF_6P.om_6P  BeginIndexSearchUsingPreviousIndexResult=on  Table=Parameter.Control.cIPC.PSM0_NF_6P.b_1  ExtrapMethod=Clip  InternalRulePriority=Speed  RndMeth=Simplest
  1-D Lookup Table2 : Lookup_n-D  NumberOfTableDimensions=1  BreakpointsForDimension1=Parameter.Control.cIPC.PSM0_NF_6P.om_6P  BeginIndexSearchUsingPreviousIndexResult=on  Table=Parameter.Control.cIPC.PSM0_NF_6P.b_0  ExtrapMethod=Clip  InternalRulePriority=Speed  RndMeth=Simplest
  Mux : Mux  Inputs=3
  b : Outport  VectorParamsAs1DForOutWhenUnconnected=off
  wires:
  1-D Lookup Table2/1 -> Mux/3
  rot speed (rad/s)/1 -> 1-D Lookup Table1/1, 1-D Lookup Table/1, 1-D Lookup Table2/1
  Mux/1 -> b/1
  1-D Lookup Table1/1 -> Mux/2
  1-D Lookup Table/1 -> Mux/1

== system ROSCO/Monitor2/Cyclic Pitch controller/2P Cyclic Pitch Controller2/M0 Signal Proc.1/Moving 1P Notch Man/Moving 1P Filt Manual/Den LPV ==
  rot speed (rad/s) : Inport
  1-D Lookup Table : Lookup_n-D  NumberOfTableDimensions=1  BreakpointsForDimension1=Parameter.Control.cIPC.PSM0_NF_1P.om_1P  BeginIndexSearchUsingPreviousIndexResult=on  Table=Parameter.Control.cIPC.PSM0_NF_1P.a_2  ExtrapMethod=Clip  InternalRulePriority=Speed  RndMeth=Simplest
  1-D Lookup Table1 : Lookup_n-D  NumberOfTableDimensions=1  BreakpointsForDimension1=Parameter.Control.cIPC.PSM0_NF_1P.om_1P  BeginIndexSearchUsingPreviousIndexResult=on  Table=Parameter.Control.cIPC.PSM0_NF_1P.a_1  ExtrapMethod=Clip  InternalRulePriority=Speed  RndMeth=Simplest
  1-D Lookup Table2 : Lookup_n-D  NumberOfTableDimensions=1  BreakpointsForDimension1=Parameter.Control.cIPC.PSM0_NF_1P.om_1P  BeginIndexSearchUsingPreviousIndexResult=on  Table=Parameter.Control.cIPC.PSM0_NF_1P.a_0  ExtrapMethod=Clip  InternalRulePriority=Speed  RndMeth=Simplest
  Mux : Mux  Inputs=3
  a : Outport  VectorParamsAs1DForOutWhenUnconnected=off
  wires:
  1-D Lookup Table2/1 -> Mux/3
  rot speed (rad/s)/1 -> 1-D Lookup Table1/1, 1-D Lookup Table/1, 1-D Lookup Table2/1
  Mux/1 -> a/1
  1-D Lookup Table1/1 -> Mux/2
  1-D Lookup Table/1 -> Mux/1

== system ROSCO/Monitor2/Cyclic Pitch controller/2P Cyclic Pitch Controller2/M0 Signal Proc.1/Moving 1P Notch Man/Moving 1P Filt Manual/Num LPV ==
  rot speed (rad/s) : Inport
  1-D Lookup Table : Lookup_n-D  NumberOfTableDimensions=1  BreakpointsForDimension1=Parameter.Control.cIPC.PSM0_NF_1P.om_1P  BeginIndexSearchUsingPreviousIndexResult=on  Table=Parameter.Control.cIPC.PSM0_NF_1P.b_2  ExtrapMethod=Clip  InternalRulePriority=Speed  RndMeth=Simplest
  1-D Lookup Table1 : Lookup_n-D  NumberOfTableDimensions=1  BreakpointsForDimension1=Parameter.Control.cIPC.PSM0_NF_1P.om_1P  BeginIndexSearchUsingPreviousIndexResult=on  Table=Parameter.Control.cIPC.PSM0_NF_1P.b_1  ExtrapMethod=Clip  InternalRulePriority=Speed  RndMeth=Simplest
  1-D Lookup Table2 : Lookup_n-D  NumberOfTableDimensions=1  BreakpointsForDimension1=Parameter.Control.cIPC.PSM0_NF_1P.om_1P  BeginIndexSearchUsingPreviousIndexResult=on  Table=Parameter.Control.cIPC.PSM0_NF_1P.b_0  ExtrapMethod=Clip  InternalRulePriority=Speed  RndMeth=Simplest
  Mux : Mux  Inputs=3
  b : Outport  VectorParamsAs1DForOutWhenUnconnected=off
  wires:
  1-D Lookup Table/1 -> Mux/1
  1-D Lookup Table1/1 -> Mux/2
  Mux/1 -> b/1
  rot speed (rad/s)/1 -> 1-D Lookup Table2/1, 1-D Lookup Table/1, 1-D Lookup Table1/1
  1-D Lookup Table2/1 -> Mux/3

== system ROSCO/Monitor2/Cyclic Pitch controller/2P Cyclic Pitch Controller2/M0 Signal Proc.1/Moving 3P Notch Man/Moving 3P Filt Manual/Den LPV ==
  rot speed (rad/s) : Inport
  1-D Lookup Table : Lookup_n-D  NumberOfTableDimensions=1  BreakpointsForDimension1=Parameter.Control.cIPC.PSM0_NF_3P.om_3P  BeginIndexSearchUsingPreviousIndexResult=on  Table=Parameter.Control.cIPC.PSM0_NF_3P.a_2  ExtrapMethod=Clip  InternalRulePriority=Speed  RndMeth=Simplest
  1-D Lookup Table1 : Lookup_n-D  NumberOfTableDimensions=1  BreakpointsForDimension1=Parameter.Control.cIPC.PSM0_NF_3P.om_3P  BeginIndexSearchUsingPreviousIndexResult=on  Table=Parameter.Control.cIPC.PSM0_NF_3P.a_1  ExtrapMethod=Clip  InternalRulePriority=Speed  RndMeth=Simplest
  1-D Lookup Table2 : Lookup_n-D  NumberOfTableDimensions=1  BreakpointsForDimension1=Parameter.Control.cIPC.PSM0_NF_3P.om_3P  BeginIndexSearchUsingPreviousIndexResult=on  Table=Parameter.Control.cIPC.PSM0_NF_3P.a_0  ExtrapMethod=Clip  InternalRulePriority=Speed  RndMeth=Simplest
  Mux : Mux  Inputs=3
  a : Outport  VectorParamsAs1DForOutWhenUnconnected=off
  wires:
  1-D Lookup Table/1 -> Mux/1
  1-D Lookup Table1/1 -> Mux/2
  Mux/1 -> a/1
  rot speed (rad/s)/1 -> 1-D Lookup Table2/1, 1-D Lookup Table/1, 1-D Lookup Table1/1
  1-D Lookup Table2/1 -> Mux/3

== system ROSCO/Monitor2/Cyclic Pitch controller/2P Cyclic Pitch Controller2/M0 Signal Proc.1/Moving 3P Notch Man/Moving 3P Filt Manual/Num LPV ==
  rot speed (rad/s) : Inport
  1-D Lookup Table : Lookup_n-D  NumberOfTableDimensions=1  BreakpointsForDimension1=Parameter.Control.cIPC.PSM0_NF_3P.om_3P  BeginIndexSearchUsingPreviousIndexResult=on  Table=Parameter.Control.cIPC.PSM0_NF_3P.b_2  ExtrapMethod=Clip  InternalRulePriority=Speed  RndMeth=Simplest
  1-D Lookup Table1 : Lookup_n-D  NumberOfTableDimensions=1  BreakpointsForDimension1=Parameter.Control.cIPC.PSM0_NF_3P.om_3P  BeginIndexSearchUsingPreviousIndexResult=on  Table=Parameter.Control.cIPC.PSM0_NF_3P.b_1  ExtrapMethod=Clip  InternalRulePriority=Speed  RndMeth=Simplest
  1-D Lookup Table2 : Lookup_n-D  NumberOfTableDimensions=1  BreakpointsForDimension1=Parameter.Control.cIPC.PSM0_NF_3P.om_3P  BeginIndexSearchUsingPreviousIndexResult=on  Table=Parameter.Control.cIPC.PSM0_NF_3P.b_0  ExtrapMethod=Clip  InternalRulePriority=Speed  RndMeth=Simplest
  Mux : Mux  Inputs=3
  b : Outport  VectorParamsAs1DForOutWhenUnconnected=off
  wires:
  1-D Lookup Table2/1 -> Mux/3
  rot speed (rad/s)/1 -> 1-D Lookup Table1/1, 1-D Lookup Table/1, 1-D Lookup Table2/1
  Mux/1 -> b/1
  1-D Lookup Table1/1 -> Mux/2
  1-D Lookup Table/1 -> Mux/1

== matlab function ROSCO/PitchSaturation/Variable Saturator1 ==
  data: pitchCommand input; lowerLimit input; pitchCommandOut output; upperLimit input; atLimit output
function [pitchCommandOut,atLimit] = variableSat(pitchCommand,lowerLimit,upperLimit)
%#codegen

if pitchCommand < lowerLimit
    pitchCommandOut = lowerLimit;
    atLimit          = 1;
    
elseif pitchCommand > upperLimit
    pitchCommandOut = upperLimit;
    atLimit         = 1;
    
else
    pitchCommandOut = pitchCommand;
    atLimit         = 0;
end

== matlab function ROSCO/BldPitch Controller/Pitch GS ==
  data: Ki output size=1; Beta input; Kp_pc input; Kp output size=1; Ki_pc input; PC_beta input
function [Ki, Kp] = GainSchedule(Beta, Kp_pc, Ki_pc,  PC_beta)

% This function calculates the current gains for a Collective Blade Pitch 
% controller
%
% Inputs: v - Current wind speed estimate, m/s.
%         ContParam - Structure of control parameters, output from
%                     ControlParameters.m
%
% Outputs: Kp - Proportional Gain
%          Ki - Integral Gain
%
% Nikhar Abbas - May 2019


%% Linear Gain Schedule
% pKp_pc = ContParam.GS.pKp_pc;
% pKi_pc = ContParam.GS.pKi_pc;
% 
% %%
% Kp = pKp_pc(1)*Beta + pKp_pc(2);
% Ki = pKi_pc(1)*Beta + pKi_pc(2);
% % Kp = pKp_pc(1)*v + pKp_pc(2)
% % Ki = pKi_pc(1)*v + pKi_pc(2);
% 
% Kpmax = pKp_pc(1)*15*pi/180 + pKp_pc(2);
% Kimax = pKi_pc(1)*15*pi/180 + pKi_pc(2);
% 
% Kp = min(Kp, Kpmax);
% Ki = min(Ki,Kimax);

%% nonlinear Gain Schedule
% Kp_pc   = R.PC_GS_KP;
% Ki_pc   = R.PC_GS_KI;
% PC_beta = R.PC_GS_angles;

beta    = max(min(Beta,PC_beta(end)), PC_beta(1));

% gains
Kp      = interp1(PC_beta,Kp_pc, beta);
Ki      = interp1(PC_beta,Ki_pc, beta);



end

== matlab function ROSCO/LinearModel_Simulink/MATLAB Function ==
  data: Azimuth input; y output; n_FixFrameOutputs input; n_RotTripletOutputs input; new_seq_out input; y_dq input
function y  = iTransverse_y(Azimuth, n_FixFrameOutputs, n_RotTripletOutputs, new_seq_out, y_dq)

% compute azimuth positions of blades:
az = Azimuth*pi/180.0 + 2*pi/3* (0:(3-1)) ; % Eq. 1, azimuth in radians   3个叶片的方位角（弧度），叶片1的方位角为初始方位角

% compute transformation matrices
cos_col = cos(az(:));  % 列向量
sin_col = sin(az(:));

tt  = [ones(3,1), cos_col, sin_col];        % Eq. 9, t_tilde


T1o = zeros(n_FixFrameOutputs+3*n_RotTripletOutputs, n_FixFrameOutputs+3*n_RotTripletOutputs);

T1o(1:n_FixFrameOutputs, 1:n_FixFrameOutputs) = eye(n_FixFrameOutputs);              % Tlo (Eq. 23)  输出相关

for ii = 1:n_RotTripletOutputs
    T1o(n_FixFrameOutputs+1+(ii-1)*3 : n_FixFrameOutputs+ii*3, n_FixFrameOutputs+1+(ii-1)*3 : n_FixFrameOutputs+ii*3) = tt;
end

y = y_dq .* 0;
y(new_seq_out, :) = T1o * y_dq(new_seq_out);

end

== matlab function ROSCO/LinearModel_Simulink/KalmanStateObserver/KalmanSP ==
  data: Am input; X_pred output; Bm input; Bmd input; X_obs input; delta_udq input; delta_wdq input
function X_pred = KalmanSP(Am, Bm, Bmd, X_obs, delta_udq, delta_wdq)
    persistent x_hat
    persistent P

    if isempty(x_hat)
        x_hat = zeros(22, 1);
        P = eye(22);
    end

    H = zeros(22, 22);  % 量测状态矩阵
    % 选择可量测量
    H(1, 1) = 1; 
    H(2, 2) = 1; 
    H(9, 9) = 1;
    H(10, 10) = 1;
    H(11, 11) = 1;
    H(18, 18) = 1;  % GenSpeed
    H(19, 19) = 1;  % RotSpeed


    Q = 1 * eye(22);     % 过程噪声协方差矩阵
    Q(20, 20) = 100;
    Q(21, 21) = 100;
    Q(22, 22) = 100;
    R = 1e-8 * eye(22);  % 观测噪声协方差
    
    v = sqrt(R) * ones(22, 1) * randn;
    z  = H * X_obs + v;
    
    % 时间更新（预测）
    x_hat_ = Am * x_hat + Bm * delta_udq + Bmd * delta_wdq;
    P_ = Am * P * Am' + Q;

    % 测量更新（校正）
    K = P_ * H' * (H * P_ * H' + R)^(-1);
    P = (eye(22) - K * H) * P_;

    x_hat = x_hat_ + K * (z - H * x_hat_);

    X_pred = x_hat;



end

== matlab function ROSCO/LinearModel_Simulink/KalmanStateObserver/Extend X_obs_Fcn ==
  data: QD_TFA1 input; X_obs output; Q_TFA1 input; QD_TSS1 input; Q_TSS1 input; RotSpeed input; ydq input
function X_obs = X_obs_Fcn(QD_TFA1, Q_TFA1, QD_TSS1, Q_TSS1, RotSpeed, ydq)
    % 需要对x进行MBC变换，但由于观测量都处于固定坐标系中，故无需进行变换
    % X为增广状态，参考文献"基于模型预测控制的大型海上风电机组降载控制"4.4.1节公式(4-28)
    persistent x_km1
    if isempty(x_km1)
        x_km1 = zeros(17, 1);
        x_km1(9, 1) = QD_TFA1;
        x_km1(1, 1) = Q_TFA1;
        x_km1(10, 1) = QD_TSS1;
        x_km1(2, 1) = Q_TSS1;
        x_km1(11, 1) = RotSpeed;
    end
    
    x_k = zeros(17, 1);
    x_k(9, 1) = QD_TFA1;
    x_k(1, 1) = Q_TFA1;
    x_k(10, 1) = QD_TSS1;
    x_k(2, 1) = Q_TSS1;
    x_k(11, 1) = RotSpeed;
    
    % 计算差分量
    delta_x_k = zeros(17, 1);
    delta_x_k(9, 1) = x_k(9, 1) - x_km1(9, 1);
    delta_x_k(1, 1) = x_k(1, 1) - x_km1(1, 1);
    delta_x_k(10, 1) = x_k(10, 1) - x_km1(10, 1);
    delta_x_k(2, 1) = x_k(2, 1) - x_km1(2, 1);
    delta_x_k(11, 1) = x_k(11, 1) - x_km1(11, 1);
    
    % 生成增广状态变量
    X_obs = zeros(17+5, 1);
    X_obs(1:17, 1) = delta_x_k;
    X_obs(18:22, 1) = ydq;

    % ----------------
    x_km1(9, 1) = x_k(9, 1);
    x_km1(1, 1) = x_k(1, 1);
    x_km1(10, 1) = x_k(10, 1);
    x_km1(2, 1) = x_k(2, 1);
    x_km1(11, 1) = x_k(11, 1);

    

end

== matlab function ROSCO/LinearModel_Simulink/KalmanStateObserver/MATLAB Function1 ==
  data: Azimuth input; ydq output; n_FixFrameOutputs input; n_RotTripletOutputs input; new_seq_out input; y input
function ydq  = Transverse_y(Azimuth, n_FixFrameOutputs, n_RotTripletOutputs, new_seq_out, y)

% compute azimuth positions of blades:
az = Azimuth*pi/180.0 + 2*pi/3* (0:(3-1)) ; % Eq. 1, azimuth in radians   3个叶片的方位角（弧度），叶片1的方位角为初始方位角

% compute transformation matrices
cos_col = cos(az(:));  % 列向量
sin_col = sin(az(:));

ttv = get_tt_inverse(sin_col, cos_col);     % inverse of tt (computed analytically in function below) 逆矩阵

T1ov = zeros(n_FixFrameOutputs+3*n_RotTripletOutputs, n_FixFrameOutputs+3*n_RotTripletOutputs);

T1ov(1:n_FixFrameOutputs, 1:n_FixFrameOutputs) = eye(n_FixFrameOutputs);              % Tlo (Eq. 23)  输出相关

for ii = 1:n_RotTripletOutputs
    T1ov(n_FixFrameOutputs+1+(ii-1)*3 : n_FixFrameOutputs+ii*3, n_FixFrameOutputs+1+(ii-1)*3 : n_FixFrameOutputs+ii*3) = ttv;
end

ydq = y .* 0;
ydq(new_seq_out, :) = T1ov * y(new_seq_out);

end





function [ttv] = get_tt_inverse(sin_col, cos_col)

    c1 = cos_col(1);
    c2 = cos_col(2);
    c3 = cos_col(3);
    
    s1 = sin_col(1);
    s2 = sin_col(2);
    s3 = sin_col(3);

    
    ttv = [ c2*s3 - s2*c3,  c3*s1 - s3*c1, c1*s2 - s1*c2
               s2 - s3 ,       s3 - s1,       s1 - s2
               c3 - c2 ,       c1 - c3,       c2 - c1 ] / (1.5*sqrt(3));

    return
end

== matlab function ROSCO/LinearModel_Simulink/KalmanStateObserver/Extend X_obs_Fcn1 ==
  data: QD_TFA1 input; X_obs output; Q_TFA1 input; QD_TSS1 input; Q_TSS1 input; RotSpeed input; Q_BNF1 input; Q_BNE1 input; QD_BNF1 input; QD_BNE1 input; ydq input
function X_obs = X_obs_Fcn1(QD_TFA1, Q_TFA1, QD_TSS1, Q_TSS1, RotSpeed, Q_BNF1, Q_BNE1, QD_BNF1, QD_BNE1, ydq)
    % 需要对x进行MBC变换，但由于观测量都处于固定坐标系中，故无需进行变换
    % X为增广状态，参考文献"基于模型预测控制的大型海上风电机组降载控制"4.4.1节公式(4-28)
    persistent x_km1
    if isempty(x_km1)
        x_km1 = zeros(17, 1);
        x_km1(9, 1) = QD_TFA1;
        x_km1(1, 1) = Q_TFA1;
        x_km1(10, 1) = QD_TSS1;
        x_km1(2, 1) = Q_TSS1;
        x_km1(11, 1) = RotSpeed;
        x_km1(3:5, 1) = Q_BNF1;
        x_km1(6:8, 1) = Q_BNE1;
        x_km1(12:14, 1) = QD_BNF1;
        x_km1(15:17, 1) = QD_BNE1;
    end
    
    x_k = zeros(17, 1);
    x_k(9, 1) = QD_TFA1;
    x_k(1, 1) = Q_TFA1;
    x_k(10, 1) = QD_TSS1;
    x_k(2, 1) = Q_TSS1;
    x_k(11, 1) = RotSpeed;
    x_k(3:5, 1) = Q_BNF1;
    x_k(6:8, 1) = Q_BNE1;
    x_k(12:14, 1) = QD_BNF1;
    x_k(15:17, 1) = QD_BNE1;
    
    % 计算差分量
    delta_x_k = zeros(17, 1);
    delta_x_k(9, 1) = x_k(9, 1) - x_km1(9, 1);
    delta_x_k(1, 1) = x_k(1, 1) - x_km1(1, 1);
    delta_x_k(10, 1) = x_k(10, 1) - x_km1(10, 1);
    delta_x_k(2, 1) = x_k(2, 1) - x_km1(2, 1);
    delta_x_k(11, 1) = x_k(11, 1) - x_km1(11, 1);
    delta_x_k(3:5, 1) = x_k(3:5, 1) - x_km1(3:5, 1);
    delta_x_k(6:8, 1) = x_k(6:8, 1) - x_km1(6:8, 1);
    delta_x_k(12:14, 1) = x_k(12:14, 1) - x_km1(12:14, 1);
    delta_x_k(15:17, 1) = x_k(15:17, 1) - x_km1(15:17, 1);
    
    % 生成增广状态变量
    X_obs = zeros(17+5, 1);
    X_obs(1:17, 1) = delta_x_k;
    X_obs(18:22, 1) = ydq;

    % ----------------
    x_km1(9, 1) = x_k(9, 1);
    x_km1(1, 1) = x_k(1, 1);
    x_km1(10, 1) = x_k(10, 1);
    x_km1(2, 1) = x_k(2, 1);
    x_km1(11, 1) = x_k(11, 1);
    x_km1(3:5, 1) = x_k(3:5, 1);
    x_km1(6:8, 1) = x_k(6:8, 1);
    x_km1(12:14, 1) = x_k(12:14, 1);
    x_km1(15:17, 1) = x_k(15:17, 1);
    

end

== matlab function ROSCO/LinearModel_Simulink/KalmanStateObserver/Extend AB ==
  settings: updateMethod=DISCRETE
  data: A input; Am output; B input; C input; D input; delta_udq_in input; Bm output; Bmd output; delta_udq output; DT input; delta_wdq_in input; Bd input; Dd input; delta_wdq output
function [Am, Bm, Bmd, delta_udq, delta_wdq] = fcn(A, B, C, D, delta_udq_in, DT, delta_wdq_in, Bd, Dd )
    persistent delta_udq_in_prior
    persistent delta_wdq_in_prior
    
    if isempty(delta_udq_in_prior)
        delta_udq_in_prior = delta_udq_in;
        delta_wdq_in_prior = delta_wdq_in;
    end
    delta_udq = delta_udq_in - delta_udq_in_prior;
    delta_wdq = delta_wdq_in - delta_wdq_in_prior;
    
    dt = 0.001;
    Am = [dt * A + eye(size(A, 1)), zeros(size(A, 1), size(C, 1));
          C, eye(size(C, 1))];
    Bm = [dt * B; D];
    Bmd = [dt * Bd; Dd];
    
    % ------------------------
    delta_udq_in_prior = delta_udq_in;
    delta_wdq_in_prior = delta_wdq_in;
end

== matlab function ROSCO/LinearModel_Simulink/KalmanStateObserver/MBC ==
  data: Azimuth input; xdq output; x1 input; x2 input; x3 input
function xdq  = MBC(Azimuth, x1, x2, x3)
x = [x1; x2; x3];
% compute azimuth positions of blades:
az = Azimuth*pi/180.0 + 2*pi/3* (0:(3-1)) ; % Eq. 1, azimuth in radians   3个叶片的方位角（弧度），叶片1的方位角为初始方位角

% compute transformation matrices
cos_col = cos(az(:));  % 列向量
sin_col = sin(az(:));

ttv = get_tt_inverse(sin_col, cos_col);     % inverse of tt (computed analytically in function below) 逆矩阵

xdq = x .* 0;
xdq = ttv * x;

end





function [ttv] = get_tt_inverse(sin_col, cos_col)

    c1 = cos_col(1);
    c2 = cos_col(2);
    c3 = cos_col(3);
    
    s1 = sin_col(1);
    s2 = sin_col(2);
    s3 = sin_col(3);

    
    ttv = [ c2*s3 - s2*c3,  c3*s1 - s3*c1, c1*s2 - s1*c2
               s2 - s3 ,       s3 - s1,       s1 - s2
               c3 - c2 ,       c1 - c3,       c2 - c1 ] / (1.5*sqrt(3));

    return
end
